simulink model "Linear_heli_model_estimator_PID"  (R2017a)
settings: Solver=ode4  StartTime=0.0  StopTime=inf  FixedStep=0.1  RelTol=1e-3
values from neighbouring files (symbols this model uses):
  Ac = [  0,0,1,0 ... (first row only)    [Linear_estimator.m]    (also in Linear_estimator_integrator.m; Linear_script_estimator.m = [Ac1,Ac2])
  Bc = [  0,0 ... (first row only)    [Linear_estimator.m]    (also in Linear_estimator_integrator.m; Linear_script_estimator.m = [0,0;0,0;Kpp/J1,-Kpy/J1;Kyp/J2,-Kyy/J2])
  Cc = [  1,0,0,0 ... (first row only)    [Linear_estimator.m]    (also in Linear_estimator_integrator.m; Linear_script_estimator.m = [1,0,0,0;0,1,0,0])
  psi_op = pi/2    (= 1.57079632679)    [Linear_estimator.m]    (also in Linear_estimator_integrator.m; Linear_script_estimator.m)
  theta_op = (-10*pi)/180    (= -0.174532925199)    [Linear_estimator.m]    (also in Linear_estimator_integrator.m; Linear_script_estimator.m)
  Vmp_op = (Kyy*mheli*g*cos(theta_op)*lcm)/(Kyy*Kpp-Kyp*Kpy)    [Linear_estimator.m]    (also in Linear_estimator_integrator.m; Linear_script_estimator.m)
  Vmy_op = (Kyp*Vmp_op)/Kyy    [Linear_estimator.m]    (also in Linear_estimator_integrator.m; Linear_script_estimator.m)
  w_psi_op = 0    [Linear_estimator.m]    (also in Linear_estimator_integrator.m; Linear_script_estimator.m)
  w_theta_op = 0    [Linear_estimator.m]    (also in Linear_estimator_integrator.m; Linear_script_estimator.m)
undefined symbols (not defined in the file or in its folder): L
libraries: simulink x2, realtime_pacer_lib x1
settings Model: Creator=ShingWai  LastModifiedBy=ShingWai

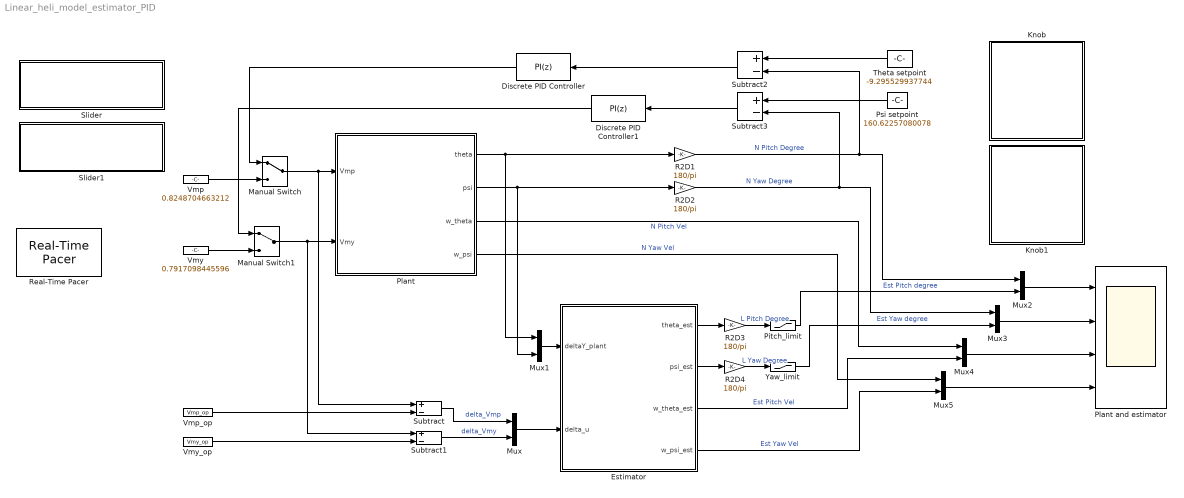
== system Linear_heli_model_estimator_PID ==
  Discrete PID Controller : simulink/Continuous/PID Controller  Controller=PI  TimeDomain=Discrete-time  SampleTime=-1  IntegratorMethod=Forward Euler  FilterMethod=Forward Euler  Form=Parallel  UseFilter=on  ControllerParametersSource=internal  P=0  I=0.000907573361479579  D=0.0132997774455979  N=30.9531371143485  InitialConditionSource=internal  InitialConditionForIntegrator=0  InitialConditionForFilter=0  ExternalReset=none  LimitOutput=on  UpperSaturationLimit=2  LowerSaturationLimit=0  LinearizeAsGain=off  AntiWindupMode=clamping  Kb=1  TrackingMode=off  Kt=1  PParamMin=[]  PParamMax=[]  IParamMin=[]  IParamMax=[]  DParamMin=[]  DParamMax=[]  NParamMin=[]  NParamMax=[]  KbParamMin=[]  KbParamMax=[]  KtParamMin=[]  KtParamMax=[]  POutMin=[]  POutMax=[]  IOutMin=[]  IOutMax=[]  DOutMin=[]  DOutMax=[]  NOutMin=[]  NOutMax=[]  KbOutMin=[]  KbOutMax=[]  KtOutMin=[]  KtOutMax=[]  IntegratorOutMin=[]  IntegratorOutMax=[]  FilterOutMin=[]  FilterOutMax=[]  SumOutMin=[]  SumOutMax=[]  SumI1OutMin=[]  SumI1OutMax=[]  SumI2OutMin=[]  SumI2OutMax=[]  SumI3OutMin=[]  SumI3OutMax=[]  SumDOutMin=[]  SumDOutMax=[]  SaturationOutMin=[]  SaturationOutMax=[]  IntegratorContinuousStateAttributes=''  IntegratorStateMustResolveToSignalObject=off  IntegratorRTWStateStorageClass=Auto  FilterContinuousStateAttributes=''  FilterStateMustResolveToSignalObject=off  FilterRTWStateStorageClass=Auto  DifferentiatorICPrevScaledInput=0  DifferentiatorOutMin=[]  DifferentiatorOutMax=[]  InitialConditionSetting=State (most efficient)
  Discrete PID Controller1 : simulink/Continuous/PID Controller  Controller=PI  TimeDomain=Discrete-time  SampleTime=-1  IntegratorMethod=Forward Euler  FilterMethod=Forward Euler  Form=Parallel  UseFilter=on  ControllerParametersSource=internal  P=-0.0211292479754596  I=-0.00097032283605342  D=-0.0494385294991883  N=316.412826035343  InitialConditionSource=internal  InitialConditionForIntegrator=0  InitialConditionForFilter=0  ExternalReset=none  LimitOutput=on  UpperSaturationLimit=2  LowerSaturationLimit=0  LinearizeAsGain=off  AntiWindupMode=clamping  Kb=1  TrackingMode=off  Kt=1  PParamMin=[]  PParamMax=[]  IParamMin=[]  IParamMax=[]  DParamMin=[]  DParamMax=[]  NParamMin=[]  NParamMax=[]  KbParamMin=[]  KbParamMax=[]  KtParamMin=[]  KtParamMax=[]  POutMin=[]  POutMax=[]  IOutMin=[]  IOutMax=[]  DOutMin=[]  DOutMax=[]  NOutMin=[]  NOutMax=[]  KbOutMin=[]  KbOutMax=[]  KtOutMin=[]  KtOutMax=[]  IntegratorOutMin=[]  IntegratorOutMax=[]  FilterOutMin=[]  FilterOutMax=[]  SumOutMin=[]  SumOutMax=[]  SumI1OutMin=[]  SumI1OutMax=[]  SumI2OutMin=[]  SumI2OutMax=[]  SumI3OutMin=[]  SumI3OutMax=[]  SumDOutMin=[]  SumDOutMax=[]  SaturationOutMin=[]  SaturationOutMax=[]  IntegratorContinuousStateAttributes=''  IntegratorStateMustResolveToSignalObject=off  IntegratorRTWStateStorageClass=Auto  FilterContinuousStateAttributes=''  FilterStateMustResolveToSignalObject=off  FilterRTWStateStorageClass=Auto  DifferentiatorICPrevScaledInput=0  DifferentiatorOutMin=[]  DifferentiatorOutMax=[]  InitialConditionSetting=State (most efficient)
  Estimator : Subsystem
  Knob : Subsystem  DialogController=hmiCreateDDGDialog  IsWebBlock=on  mask(MWDashboardBlock){webBlockId=f7d6c496-e7f3-45e5-b299-ebdecf5f4c4e, webBlockType=continuousknob, ShowInLibBrowser=on, ShowInitialText=on, HMISrcModelName=Linear_heli_model_estimator_PID}
      mask prompts: webBlockId "WebBlock Id"; webBlockType "WebBlock Type"; HMISrcModelName "Source Model"
      mask help: SimulinkHMI:dialogs:ContinuousKnobDialogDesc
      mask Help: helpview([docroot '/mapfiles/simulink.map'], 'hmi_knob')
      mask Display:
      | if strcmp(get_param(bdroot(gcb),'BlockDiagramType'), 'library')
      |     image([(matlabroot) '/toolbox/simulink/hmi/icons/ContinuousKnob.png']);
      | end
  Knob1 : Subsystem  DialogController=hmiCreateDDGDialog  IsWebBlock=on  mask(MWDashboardBlock){webBlockId=7ec695cf-c3d5-415a-ba20-dfe3f8e66350, webBlockType=continuousknob, ShowInLibBrowser=on, ShowInitialText=on, HMISrcModelName=Linear_heli_model_estimator_PID}
      mask prompts: webBlockId "WebBlock Id"; webBlockType "WebBlock Type"; HMISrcModelName "Source Model"
      mask help: SimulinkHMI:dialogs:ContinuousKnobDialogDesc
      mask Help: helpview([docroot '/mapfiles/simulink.map'], 'hmi_knob')
      mask Display:
      | if strcmp(get_param(bdroot(gcb),'BlockDiagramType'), 'library')
      |     image([(matlabroot) '/toolbox/simulink/hmi/icons/ContinuousKnob.png']);
      | end
  Manual Switch : ManualSwitch
  Manual Switch1 : ManualSwitch
  Mux{,1..5} (6 alike) : Mux  Inputs=2
  Pitch_limit : Saturate  UpperLimit=45  LowerLimit=-45  LinearizeAsGain=off
  Plant : Subsystem
  Plant and estimator : Scope  NumInputPorts=4
  Psi setpoint : Constant  Value=160.62257080078
  R2D{1..4} (4 alike) : Gain  Gain=180/pi
  Real-Time Pacer : realtime_pacer_lib/Real-Time Pacer  simTimePerRealTime=5
  Slider : Subsystem  DialogController=hmiCreateDDGDialog  IsWebBlock=on  mask(MWDashboardBlock){webBlockId=ee768af0-5787-424b-83ad-de7ba901ce7c, webBlockType=slider, ShowInLibBrowser=on, ShowInitialText=on, HMISrcModelName=Linear_heli_model_estimator_PID}
      mask prompts: webBlockId "WebBlock Id"; webBlockType "WebBlock Type"; HMISrcModelName "Source Model"
      mask help: SimulinkHMI:dialogs:SliderDialogDesc
      mask Help: helpview([docroot '/mapfiles/simulink.map'], 'hmi_slider')
      mask Display:
      | if strcmp(get_param(bdroot(gcb),'BlockDiagramType'), 'library')
      |     image([(matlabroot) '/toolbox/simulink/hmi/icons/Slider.png']);
      | end
  Slider1 : Subsystem  DialogController=hmiCreateDDGDialog  IsWebBlock=on  mask(MWDashboardBlock){webBlockId=fc4e30f5-1f0f-4f3d-9211-693a563b3a2e, webBlockType=slider, ShowInLibBrowser=on, ShowInitialText=on, HMISrcModelName=Linear_heli_model_estimator_PID}
      mask prompts: webBlockId "WebBlock Id"; webBlockType "WebBlock Type"; HMISrcModelName "Source Model"
      mask help: SimulinkHMI:dialogs:SliderDialogDesc
      mask Help: helpview([docroot '/mapfiles/simulink.map'], 'hmi_slider')
      mask Display:
      | if strcmp(get_param(bdroot(gcb),'BlockDiagramType'), 'library')
      |     image([(matlabroot) '/toolbox/simulink/hmi/icons/Slider.png']);
      | end
  Subtract{,1..3} (4 alike) : Sum  Inputs=+-
  Theta setpoint : Constant  Value=-9.295529937744
  Vmp : Constant  Value=0.8248704663212
  Vmp_op : Constant  Value=Vmp_op
  Vmy : Constant  Value=0.7917098445596
  Vmy_op : Constant  Value=Vmy_op
  Yaw_limit : Saturate  UpperLimit=180  LowerLimit=0  LinearizeAsGain=off
  wires:
  R2D1/1 -> Subtract2/2, Mux2/1  "N Pitch Degree"
  R2D2/1 -> Subtract3/2, Mux3/1  "N Yaw Degree"
  Vmp_op/1 -> Subtract/2
  Vmy_op/1 -> Subtract1/2
  Subtract1/1 -> Mux/2  "delta_Vmy"
  Subtract/1 -> Mux/1  "delta_Vmp"
  R2D3/1 -> Pitch_limit/1  "L Pitch Degree"
  Pitch_limit/1 -> Mux2/2  "Est Pitch degree"
  R2D4/1 -> Yaw_limit/1  "L Yaw Degree"
  Yaw_limit/1 -> Mux3/2  "Est Yaw degree"
  Plant/4(w_psi) -> Mux5/1  "N Yaw Vel"
  Plant/3(w_theta) -> Mux4/1  "N Pitch Vel"
  Plant/1(theta) -> Mux1/1, R2D1/1
  Plant/2(psi) -> Mux1/2, R2D2/1
  Estimator/3(w_theta_est) -> Mux4/2  "Est Pitch Vel"
  Estimator/4(w_psi_est) -> Mux5/2  "Est Yaw Vel"
  Estimator/1(theta_est) -> R2D3/1
  Estimator/2(psi_est) -> R2D4/1
  Mux1/1 -> Estimator/1(deltaY_plant)
  Mux/1 -> Estimator/2(delta_u)
  Mux2/1 -> Plant and estimator/1
  Mux3/1 -> Plant and estimator/2
  Mux4/1 -> Plant and estimator/3
  Mux5/1 -> Plant and estimator/4
  Theta setpoint/1 -> Subtract2/1
  Psi setpoint/1 -> Subtract3/1
  Vmp/1 -> Manual Switch/2
  Manual Switch/1 -> Subtract/1, Plant/1(Vmp)
  Manual Switch1/1 -> Subtract1/1, Plant/2(Vmy)
  Vmy/1 -> Manual Switch1/2
  Subtract2/1 -> Discrete PID Controller/1
  Discrete PID Controller/1 -> Manual Switch/1
  Discrete PID Controller1/1 -> Manual Switch1/1
  Subtract3/1 -> Discrete PID Controller1/1

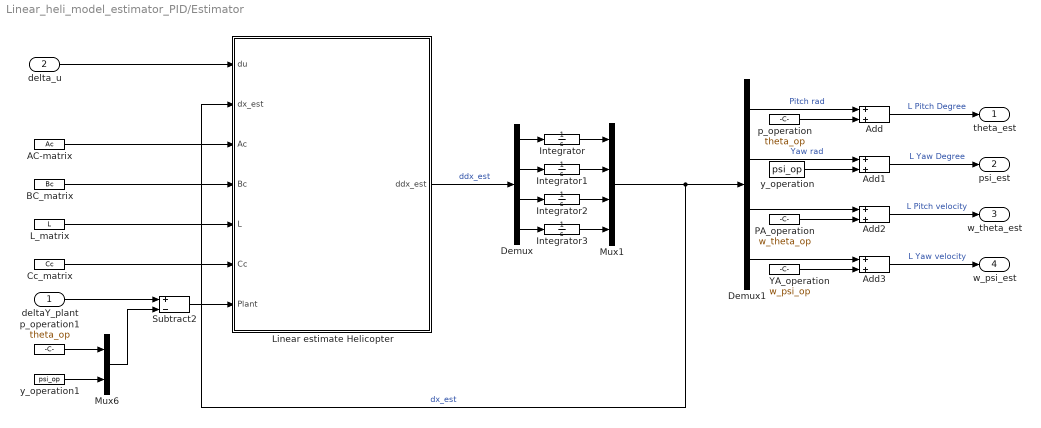
== system Linear_heli_model_estimator_PID/Estimator ==
  deltaY_plant : Inport
  delta_u : Inport  Port=2
  AC-matrix : Constant  Value=Ac
  Add{,1..3} (4 alike) : Sum
  BC_matrix : Constant  Value=Bc
  Cc_matrix : Constant  Value=Cc
  Demux : Demux
  Demux1 : Demux
  Integrator : Integrator  UpperSaturationLimit=0.9604  LowerSaturationLimit=-0.7854
  Integrator1 : Integrator  UpperSaturationLimit=pi-psi_op  LowerSaturationLimit=0-psi_op
  Integrator2 : Integrator
  Integrator3 : Integrator
  L_matrix : Constant  Value=L
  Linear estimate Helicopter : MATLAB Function  TreatAsAtomicUnit=on
  Mux1 : Mux
  Mux6 : Mux  Inputs=2
  PA_operation : Constant  Value=w_theta_op
  Subtract2 : Sum  Inputs=+-
  YA_operation : Constant  Value=w_psi_op
  p_operation : Constant  Value=theta_op
  p_operation1 : Constant  Value=theta_op  VectorParams1D=off
  y_operation : Constant  Value=psi_op
  y_operation1 : Constant  Value=psi_op  VectorParams1D=off
  theta_est : Outport
  psi_est : Outport  Port=2
  w_theta_est : Outport  Port=3
  w_psi_est : Outport  Port=4
  wires:
  AC-matrix/1 -> Linear estimate Helicopter/3(Ac)
  Linear estimate Helicopter/1(ddx_est) -> Demux/1  "ddx_est"
  BC_matrix/1 -> Linear estimate Helicopter/4(Bc)
  PA_operation/1 -> Add2/2
  Mux1/1 -> Linear estimate Helicopter/2(dx_est), Demux1/1  "dx_est"
  Demux1/2 -> Add1/1  "Yaw rad"
  Demux1/4 -> Add3/1
  Add3/1 -> w_psi_est/1  "L Yaw velocity"
  Demux1/1 -> Add/1  "Pitch rad"
  YA_operation/1 -> Add3/2
  Add2/1 -> w_theta_est/1  "L Pitch velocity"
  Add/1 -> theta_est/1  "L Pitch Degree"
  Add1/1 -> psi_est/1  "L Yaw Degree"
  p_operation/1 -> Add/2
  y_operation/1 -> Add1/2
  Demux1/3 -> Add2/1
  L_matrix/1 -> Linear estimate Helicopter/5(L)
  p_operation1/1 -> Mux6/1
  y_operation1/1 -> Mux6/2
  Mux6/1 -> Subtract2/2
  Subtract2/1 -> Linear estimate Helicopter/7(Plant)
  deltaY_plant/1 -> Subtract2/1
  delta_u/1 -> Linear estimate Helicopter/1(du)
  Cc_matrix/1 -> Linear estimate Helicopter/6(Cc)
  Demux/1 -> Integrator/1
  Integrator/1 -> Mux1/1
  Integrator1/1 -> Mux1/2
  Demux/2 -> Integrator1/1
  Integrator2/1 -> Mux1/3
  Demux/3 -> Integrator2/1
  Demux/4 -> Integrator3/1
  Integrator3/1 -> Mux1/4

== system Linear_heli_model_estimator_PID/Knob ==

== system Linear_heli_model_estimator_PID/Knob1 ==

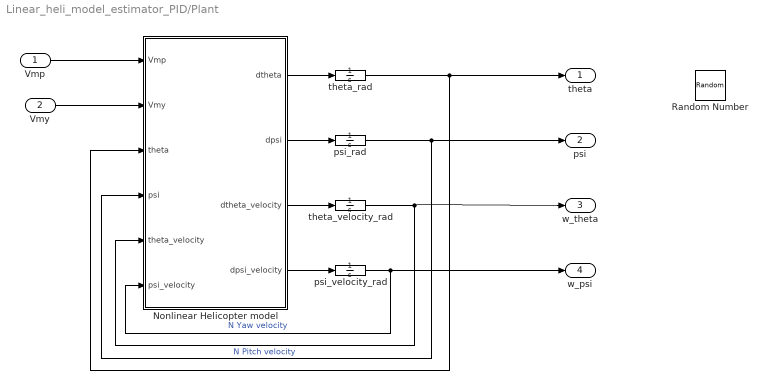
== system Linear_heli_model_estimator_PID/Plant ==
  Vmp : Inport
  Vmy : Inport  Port=2
  Nonlinear Helicopter model : MATLAB Function  TreatAsAtomicUnit=on
  Random Number : RandomNumber  Variance=0.0001
  psi_rad : Integrator  InitialCondition=psi_op  LimitOutput=on  UpperSaturationLimit=pi  LowerSaturationLimit=0
  psi_velocity_rad : Integrator  InitialCondition=w_psi_op
  theta_rad : Integrator  InitialCondition=theta_op  LimitOutput=on  UpperSaturationLimit=0.7854  LowerSaturationLimit=-0.7854
  theta_velocity_rad : Integrator  InitialCondition=w_theta_op
  theta : Outport
  psi : Outport  Port=2
  w_theta : Outport  Port=3
  w_psi : Outport  Port=4
  wires:
  Vmy/1 -> Nonlinear Helicopter model/2(Vmy)
  Vmp/1 -> Nonlinear Helicopter model/1(Vmp)
  psi_rad/1 -> psi/1, Nonlinear Helicopter model/4(psi)
  Nonlinear Helicopter model/3(dtheta_velocity) -> theta_velocity_rad/1
  psi_velocity_rad/1 -> w_psi/1, Nonlinear Helicopter model/6(psi_velocity)  "N Yaw velocity"
  theta_rad/1 -> theta/1, Nonlinear Helicopter model/3(theta)
  Nonlinear Helicopter model/4(dpsi_velocity) -> psi_velocity_rad/1
  theta_velocity_rad/1 -> w_theta/1, Nonlinear Helicopter model/5(theta_velocity)  "N Pitch velocity"
  Nonlinear Helicopter model/1(dtheta) -> theta_rad/1
  Nonlinear Helicopter model/2(dpsi) -> psi_rad/1

== system Linear_heli_model_estimator_PID/Slider ==

== system Linear_heli_model_estimator_PID/Slider1 ==

== matlab function Linear_heli_model_estimator_PID/Plant/Nonlinear Helicopter model ==
  data: Vmp input; dtheta output; Vmy input; theta input; psi input; theta_velocity input; psi_velocity input; dpsi output; dtheta_velocity output; dpsi_velocity output
function [dtheta,dpsi,dtheta_velocity,dpsi_velocity] = fcn(Vmp,Vmy,theta,psi,theta_velocity,psi_velocity)

%%Parameters of the system part 1
lcm = 0.015;    %[m]            % Distance between the pivot point and center of mass
mheli = 0.479;  %[kg]           % Total moving mass of heli
Jeqp = 0.0172; 
Jeqy= 0.0210;    %[kg/m2]       % Moment of inertia pitch and yaw axis
g = 9.81;        %[m/s2]         % Acceleration due to gravity
%%Parameter of the system part 2
Kpp = 0.0556;    %[Nm/V]         % Torque constant on pitch for pitch motor
Kyy = 0.21084;   %[Nm/V]         % Torque constant on yaw for yaw motor
Kpy = 0.005;     %[Nm/V]         % Torque constant on pitch from yaw motor
Kyp = 0.15;      %[Nm/V]         % Torque constan on pitch from pithc motor
Bp = 0.01;       %[N/V]          % Damping friction factor about pitch
By = 0.08;       %[N/V]          % Damping friction fator about yaw

%% 4 ODE
dtheta_dt = theta_velocity;
dpsi_dt = psi_velocity;
dthetaVelocity_dt = ((Kpp*Vmp)-(Kpy*Vmy)-(Bp*theta_velocity+mheli*psi_velocity^2*sin(theta)*lcm^2*cos(theta)+mheli*g*cos(theta)*lcm))/(Jeqp+mheli*lcm^2);
dpsiVelocity_dt = ((Kyp*Vmp)-(Kyy*Vmy)+(2*mheli*psi_velocity*sin(theta)*lcm^2*cos(theta)*theta_velocity)-(By*psi_velocity))/(Jeqy+mheli*cos(theta)^2*lcm^2);

%% Output
dtheta = dtheta_dt;
dpsi = dpsi_dt;
dtheta_velocity = dthetaVelocity_dt;
dpsi_velocity = dpsiVelocity_dt;

== matlab function Linear_heli_model_estimator_PID/Estimator/Linear estimate Helicopter ==
  data: du input size=[2,1]; ddx_est output size=[4,1]; dx_est input size=[4,1]; Ac input size=[4,4]; Bc input size=[4,2]; L input size=[4,2]; Cc input size=[2,4]; Plant input size=[2,1]
function ddx_est = fcn(du,dx_est,Ac,Bc, L,Cc, Plant)
%delta delta estimate = Ac*delta estimate + Bc *delta u + 
%L(delta plant - Cc *delta estimate

ddx_est=Ac*dx_est+Bc*du+L*(Plant-Cc*dx_est);
